simulink model "swGedaempftEnergie"  (R2019b)
settings: Solver=ode4  StartTime=0.0  StopTime=15.0  FixedStep=0.1  RelTol=1e-3  EnableMultiTasking=on
settings Model: Creator=Reichl  LastModifiedBy=jakob
settings DataIOCC: LimitDataPoints=on  SaveFormat=Array  SignalLoggingSaveFormat=ModelDataLogs  ReturnWorkspaceOutputs=off
settings OptimizationCC: ExpressionDepthLimit=2147483647  LifeSpan=inf
settings DebuggingCC: UnderspecifiedInitializationDetection=Classic  MergeDetectMultiDrivingBlocksExec=none  SolverPrmCheckMsg=warning  FcnCallInpInsideContextMsg=warning  StateNameClashWarn=warning  SFUnexpectedBacktrackingDiag=warning  SFNoUnconditionalDefaultTransitionDiag=warning  SFExecutionAtInitializationDiag=none  ArithmeticOperatorsInVariantConditions=warning
settings HardwareCC: ProdBitPerPointer=32  ProdBitPerSizeT=32  ProdBitPerPtrDiffT=32  ProdLargestAtomicFloat=None  ProdIntDivRoundTo=Undefined  ProdEndianess=Unspecified  ProdWordSize=32  ProdHWDeviceType=32-bit Generic
settings ModelReferenceCC: PropagateSignalLabelsOutOfModel=off
settings SFSimCC: SimUseLocalCustomCode=off  CustomCodeUndefinedFunction=UseInterfaceOnly
settings RTWCC: RTWUseLocalCustomCode=off
settings CodeAppCC: StateflowObjectComments=on
settings GRTTargetCC: TargetLangStandard=C89/C90 (ANSI)  GeneratePreprocessorConditionals=Disable all  CombineOutputUpdateFcns=off  GRTInterface=on
settings ConfigComp: CovMetricSettings=dw  CovHtmlReporting=on  CovSaveCumulativeToWorkspaceVar=on  CovSaveSingleToWorkspaceVar=on  CovExternalEMLEnable=off  CovSFcnEnable=off

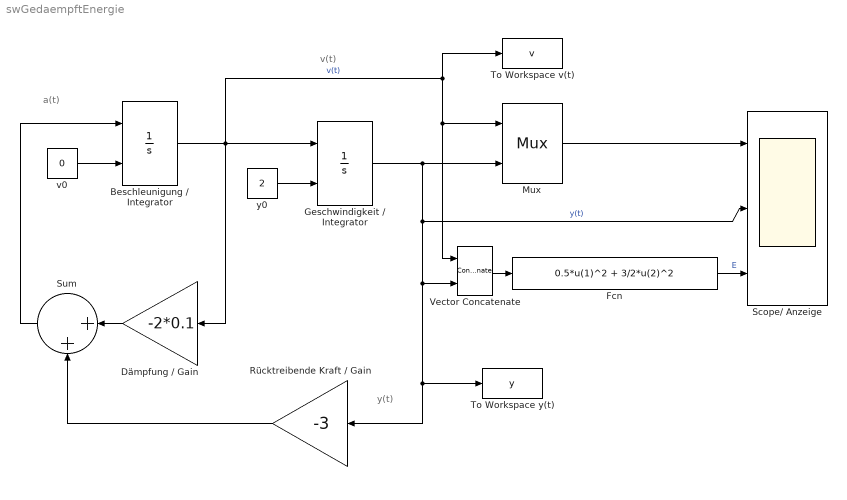
== system swGedaempftEnergie ==
  note: v(t)
  note: y(t)
  note: a(t)
  Beschleunigung / Integrator : Integrator  InitialConditionSource=external
  Dämpfung / Gain : Gain  Gain=-2*0.1
  Fcn : Fcn  Expr=0.5*u(1)^2 + 3/2*u(2)^2
  Geschwindigkeit / Integrator : Integrator  InitialConditionSource=external  InitialCondition=3
  Mux : Mux  Inputs=2
      settings: DisplayOption=signals
  Rücktreibende Kraft / Gain : Gain  Gain=-3
  Scope/ Anzeige : Scope  NumInputPorts=3
  Sum : Sum  Inputs=|++
  To Workspace v(t) : ToWorkspace  VariableName=v  SampleTime=-1
  To Workspace y(t) : ToWorkspace  VariableName=y  SampleTime=-1
  Vector Concatenate : Concatenate
  v0 : Constant  Value=0
  y0 : Constant  Value=2
  wires:
  Beschleunigung / Integrator/1 -> Geschwindigkeit / Integrator/1, To Workspace v(t)/1, Vector Concatenate/1, Mux/1, Dämpfung / Gain/1  "v(t)"
  Geschwindigkeit / Integrator/1 -> Vector Concatenate/2, To Workspace y(t)/1, Rücktreibende Kraft / Gain/1, Scope/ Anzeige/2, Mux/2  "y(t)"
  Dämpfung / Gain/1 -> Sum/1
  Rücktreibende Kraft / Gain/1 -> Sum/2
  Sum/1 -> Beschleunigung / Integrator/1
  v0/1 -> Beschleunigung / Integrator/2
  y0/1 -> Geschwindigkeit / Integrator/2
  Fcn/1 -> Scope/ Anzeige/3  "E"
  Vector Concatenate/1 -> Fcn/1
  Mux/1 -> Scope/ Anzeige/1
